simulink model "LinearizedBottom"  (R2019a)
settings: Solver=FixedStepAuto  StartTime=0.0  StopTime=10  FixedStep=0.001  RelTol=1e-3
settings Model: Creator=houte  LastModifiedBy=coeng

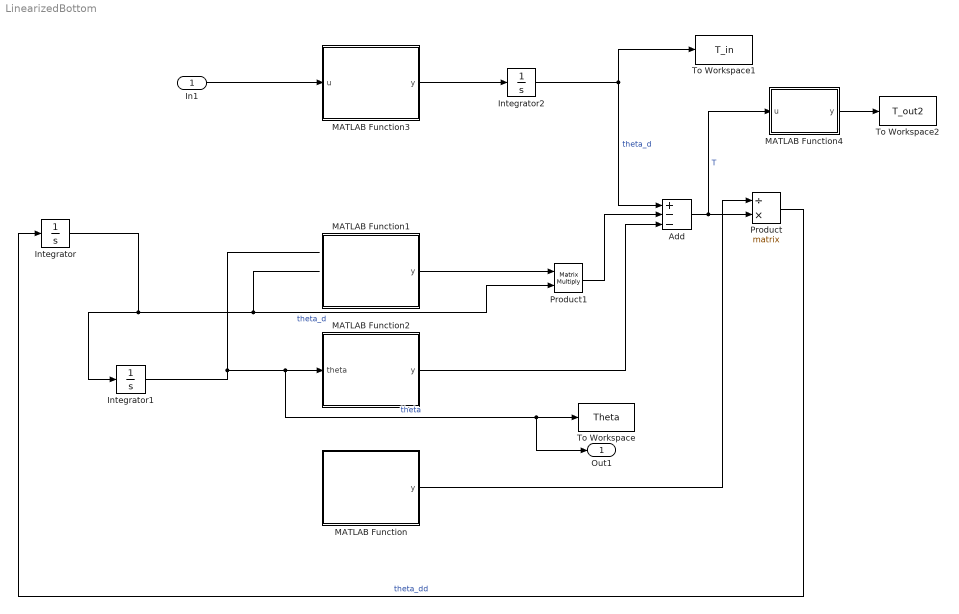
== system LinearizedBottom ==
  In1 : Inport
  Add : Sum  Inputs=+--
  Integrator : Integrator  InitialCondition=[0; 0]
  Integrator1 : Integrator  InitialCondition=firstLocation'
  Integrator2 : Integrator  InitialCondition=[0; 0]
  MATLAB Function : MATLAB Function  TreatAsAtomicUnit=on
  MATLAB Function1 : MATLAB Function  TreatAsAtomicUnit=on
  MATLAB Function2 : MATLAB Function  TreatAsAtomicUnit=on
  MATLAB Function3 : MATLAB Function  TreatAsAtomicUnit=on
  MATLAB Function4 : MATLAB Function  TreatAsAtomicUnit=on
  Product : Product  Inputs=/*  Multiplication=Matrix(*)
  Product1 : Product  Multiplication=Matrix(*)
  To Workspace : ToWorkspace  VariableName=Theta  SaveFormat=Timeseries  SampleTime=-1
  To Workspace1 : ToWorkspace  VariableName=T_in  SaveFormat=Timeseries  SampleTime=-1
  To Workspace2 : ToWorkspace  VariableName=T_out2  SaveFormat=Timeseries  SampleTime=-1
  Out1 : Outport
  wires:
  Integrator/1 -> Product1/2, Integrator1/1  "theta_d"
  Integrator1/1 -> Out1/1, To Workspace/1, MATLAB Function2/1(theta)  "theta"
  Add/1 -> MATLAB Function4/1(u), Product/2  "T"
  MATLAB Function1/1(y) -> Product1/1
  MATLAB Function3/1(y) -> Integrator2/1
  MATLAB Function2/1(y) -> Add/3
  MATLAB Function/1(y) -> Product/1
  Product/1 -> Integrator/1  "theta_dd"
  Integrator2/1 -> Add/1, To Workspace1/1  "theta_d"
  Product1/1 -> Add/2
  MATLAB Function4/1(y) -> To Workspace2/1
  In1/1 -> MATLAB Function3/1(u)

== matlab function LinearizedBottom/MATLAB Function1 ==
  data: y output; Parameters parameter
function y = C(Parameters)
y = [Parameters.b1 , 0;
    0, Parameters.b2];

== matlab function LinearizedBottom/MATLAB Function ==
  data: y output; Parameters parameter
function y = M(Parameters)

y = [Parameters.P1 + Parameters.P2 + 2*Parameters.P3, Parameters.P2 + Parameters.P3;
     Parameters.P2 + Parameters.P3, Parameters.P2];

== matlab function LinearizedBottom/MATLAB Function2 ==
  data: theta input; y output; Parameters parameter
function y = G(theta, Parameters)
    theta1 = theta(1);
    theta2 = theta(2);

y = [Parameters.g1*(theta1-pi) - Parameters.g2*(-theta2 + pi - theta1 + pi);
     -Parameters.g2*(-theta2 + pi - theta1 + pi)]

== matlab function LinearizedBottom/MATLAB Function3 ==
  data: u input; y output; Parameters parameter
function y = T(u, Parameters)
    % T = km*u - Te*dTe;
    %dTe = (km*u-T)/Te
    dTe = (Parameters.km*u)/Parameters.Te;
y = [dTe; 0];

== matlab function LinearizedBottom/MATLAB Function4 ==
  data: u input; y output
function y = fcn(u)

y = u;
